simulink model "P2_1_b_IAAC"  (R2021b)
settings: Solver=VariableStepAuto  StartTime=0.0  StopTime=100  RelTol=1e-3
settings Model: Creator=usuario_local  LastModifiedBy=Pablo
settings SolverCC: AlgebraicLoopSolver=TrustRegion
settings DebuggingCC: SFMachineParentedDataDiag=warning

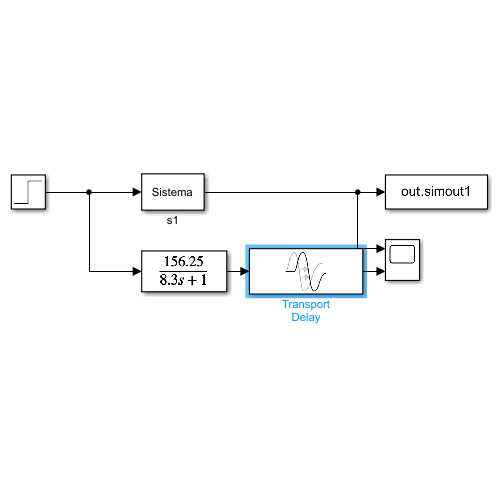
[thumbnail: Simulink's stored preview of the top-level diagram]
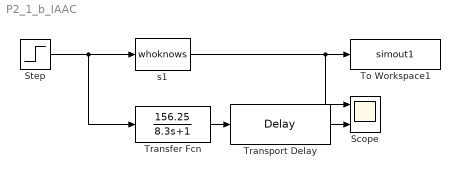
== system P2_1_b_IAAC ==
  Scope : Scope  NumInputPorts=2
  Step : Step  SampleTime=0
  To Workspace1 : ToWorkspace  VariableName=simout1  SaveFormat=Timeseries  SampleTime=-1
  Transfer Fcn : TransferFcn  Numerator=156.25  Denominator=[8.3 1]
  Transport Delay : TransportDelay  DelayTime=6
  s1 : M-S-Function  FunctionName=whoknows  Parameters=L, P1, P2, T, R  mask{L=4, P1=1, P2=1, T=1, R=0}
      mask prompts: L "Laboratorio"; P1 "Primer digito del Puesto"; P2 "Segundo digito del Puesto"; T "Tipo de Planta"; R "Ruido"
      mask Display: disp('Sistema')
  wires:
  Step/1 -> Transfer Fcn/1, s1/1
  s1/1 -> Scope/1, To Workspace1/1
  Transfer Fcn/1 -> Transport Delay/1
  Transport Delay/1 -> Scope/2
